simulink model "task1"  (R2018a)
settings: Solver=ode1  StartTime=0.0  StopTime=inf  FixedStep=0.01  RelTol=1e-3
settings Model: Creator=richardkong  LastModifiedBy=richardkong

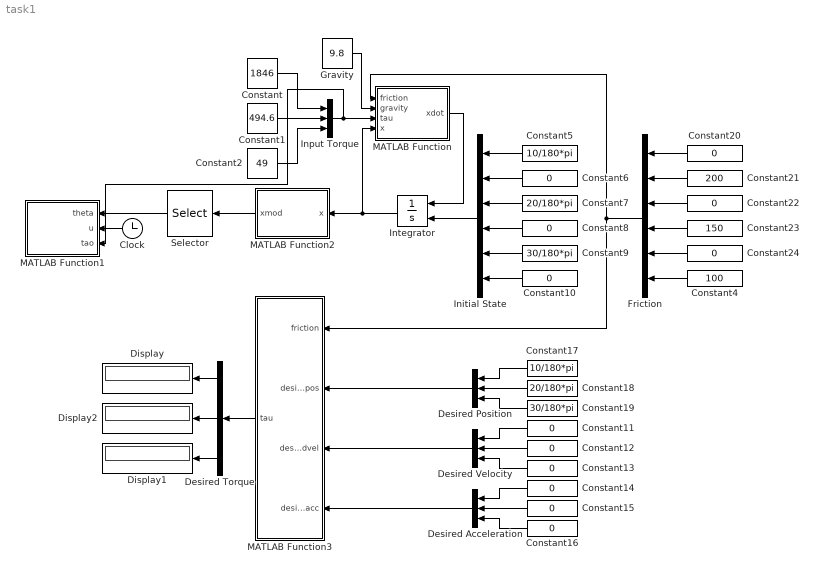
== system task1 ==
  Clock : Clock
  Constant : Constant  Value=1846
  Constant1 : Constant  Value=494.6
  Constant{6,8,10..16,20,22,24} (12 alike) : Constant  Value=0
  Constant17 : Constant  Value=10/180*pi
  Constant18 : Constant  Value=20/180*pi
  Constant19 : Constant  Value=30/180*pi
  Constant2 : Constant  Value=49
  Constant21 : Constant  Value=200
  Constant23 : Constant  Value=150
  Constant4 : Constant  Value=100
  Constant5 : Constant  Value=10/180*pi
  Constant7 : Constant  Value=20/180*pi
  Constant9 : Constant  Value=30/180*pi
  Desired Acceleration : BusCreator  Inputs=3
  Desired Position : BusCreator  Inputs=3
  Desired Torque : Demux  Outputs=3
  Desired Velocity : BusCreator  Inputs=3
  Display : Display
  Display1 : Display
  Display2 : Display
  Friction : BusCreator  Inputs=6
  Gravity : Constant  Value=9.8
  Initial State : BusCreator  Inputs=6
  Input Torque : BusCreator  Inputs=3
  Integrator : Integrator  InitialConditionSource=external  InitialCondition=[1/18*pi;0;1/9*pi;0;1/6*pi;0]
  MATLAB Function : MATLAB Function  TreatAsAtomicUnit=on
  MATLAB Function1 : MATLAB Function  TreatAsAtomicUnit=on
  MATLAB Function2 : MATLAB Function  TreatAsAtomicUnit=on
  MATLAB Function3 : MATLAB Function  TreatAsAtomicUnit=on
  Selector : Selector  InputPortWidth=6  IndexOptions=Index vector (dialog)  Indices=[1 3 5]  OutputSizes=1
  wires:
  Integrator/1 -> MATLAB Function2/1(x), MATLAB Function/4(x)
  Selector/1 -> MATLAB Function1/1(theta)
  MATLAB Function/1(xdot) -> Integrator/1
  Constant1/1 -> Input Torque/2
  Constant2/1 -> Input Torque/3
  Constant/1 -> Input Torque/1
  Input Torque/1 -> MATLAB Function1/3(tao), MATLAB Function/3(tau)
  Gravity/1 -> MATLAB Function/2(gravity)
  MATLAB Function2/1(xmod) -> Selector/1
  Friction/1 -> MATLAB Function3/1(friction), MATLAB Function/1(friction)
  Initial State/1 -> Integrator/2
  Constant5/1 -> Initial State/1
  Constant10/1 -> Initial State/6
  Constant9/1 -> Initial State/5
  Constant8/1 -> Initial State/4
  Constant7/1 -> Initial State/3
  Constant6/1 -> Initial State/2
  Constant11/1 -> Desired Velocity/1
  Constant13/1 -> Desired Velocity/3
  Constant12/1 -> Desired Velocity/2
  Constant15/1 -> Desired Acceleration/2
  Constant16/1 -> Desired Acceleration/3
  Constant14/1 -> Desired Acceleration/1
  Constant18/1 -> Desired Position/2
  Constant19/1 -> Desired Position/3
  Constant17/1 -> Desired Position/1
  MATLAB Function3/1(tau) -> Desired Torque/1
  Desired Position/1 -> MATLAB Function3/2(desiredpos)
  Desired Velocity/1 -> MATLAB Function3/3(desiredvel)
  Desired Acceleration/1 -> MATLAB Function3/4(desiredacc)
  Desired Torque/3 -> Display1/1
  Desired Torque/2 -> Display2/1
  Desired Torque/1 -> Display/1
  Constant20/1 -> Friction/1
  Constant23/1 -> Friction/4
  Constant22/1 -> Friction/3
  Constant21/1 -> Friction/2
  Constant4/1 -> Friction/6
  Constant24/1 -> Friction/5
  Clock/1 -> MATLAB Function1/2(u)

== matlab function task1/MATLAB Function1 ==
  data: theta input; u input; tao input
function animate(theta,u,tao)
%#codegen
coder.extrinsic('saveas');
coder.extrinsic('num2str');
u = int16( u / 0.01) + 1;
theta1 = theta(1);
theta2 = theta(2);
theta3 = theta(3);
%hold off
T_0 = eye(4);
hold off
l1 = 4;
l2 = 3;
l3 = 2;
point1=[[0,0,0];[4,0,0]];
point2 = [[0,0,0];[3,0,0]];
point3 = [[0,0,0];[2,0,0]];

T_01 = [cos(theta1) -sin(theta1) 0 0; sin(theta1) cos(theta1) 0 0; 0 0 1 0; 0 0 0 1];
T_12 = [cos(theta2) -sin(theta2) 0 l1; sin(theta2) cos(theta2) 0 0; 0 0 1 0; 0 0 0 1];
T_23 = [cos(theta3) -sin(theta3) 0 l2; sin(theta3) cos(theta3) 0 0; 0 0 1 0; 0 0 0 1];

point1 = [point1 [1;1]];
point2 = [point2 [1;1]];
point3 = [point3 [1;1]];
     
point1 = (T_0 * T_01 * point1')';
       
point2 = (T_0 * T_01 * T_12 * point2')';

point3 = (T_0 * T_01 * T_12 * T_23 * point3')';

plot(point1(:,1),point1(:,2));
hold on
plot(point2(:,1),point2(:,2));
grid on
plot(point3(:,1),point3(:,2));
grid on
axis([-15 15 -15 15 -15 15]);
xlabel('X');
ylabel('Y');
title(['With Torque 1 = ',num2str(tao(1)),', Torque 2 = ',num2str(tao(2)),', Torque 3 = ',num2str(tao(3)),', With Gravity']);
if rem(u, 10) == 1
    saveas(gcf,['/Users/richardkong/Desktop/Robotics/Final/Joint3/',num2str(u,'%04d')],'png');
end
end

== matlab function task1/MATLAB Function ==
  data: friction input; gravity input; tau input; xdot output; x input
function xdot = Dynamic(friction, gravity, tau, x)
%#codegen
theta1 = x(1);
theta_1 = x(2);
theta2 = x(3);
theta_2 = x(4);
theta3 = x(5);
theta_3 = x(6);

f_1 = friction(2);
f_2 = friction(4);
f_3 = friction(6);

g = gravity;
tau1 = tau(1);
tau2 = tau(2);
tau3 = tau(3);

m1 = 20;
m2 = 15;
m3 = 10;
l1 = 4;
l2 = 3;
l3 = 2;
Izz1 = 0.5;
Izz2 = 0.2;
Izz3 = 0.1;

M11 = m3 * (l1^2 + l2^2 + l3^2/4 + 2*l1*l2*cos(theta2) + l2*l3*cos(theta3) + l1*l3*cos(theta2 + theta3)) + m2 * (l1^2 + l2^2/4 + l1*l2*cos(theta2)) + m1 * l1^2/4 + Izz1 + Izz2 + Izz3;
M12 = m3 * (l2^2 + l3^2/4 + l1*l2*cos(theta2) + l2*l3*cos(theta3) + l1*l3/2*cos(theta2 + theta3)) + m2 * (l2^2/4 + l1*l2/2*cos(theta2)) + Izz2 + Izz3;
M13 = m3 * (l3^2/4 + l2*l3/2*cos(theta3) + l1*l3/2*cos(theta2 + theta3)) + Izz3;
M21 = M12;
M22 = m3 * (l2^2 + l3^2/4 + l2*l3*cos(theta3)) + m2 * l2^2/4 + Izz2 + Izz3;
M23 = m3 * (l3^2/4 + l2*l3/2*cos(theta3)) + Izz3;
M31 = M13;
M32 = M23;
M33 = m3 * l3^2/4 + Izz3;

C12 = m3 * (-l1*l2*sin(theta2) - l1*l3/2*sin(theta2 + theta3)) + m2 * (-l1*l2/2*sin(theta2));
C21 = -C12;
C13 = m3 * (-l2*l3/2*sin(theta3) - l1*l3/2*sin(theta2 + theta3));
C31 = -C13;
C23 = m3 * (-l2 * l3 / 2 * sin(theta3));
C32 = -C23;

B11 = 2 * (m3 * (-l1*l2*sin(theta2)-l1*l3/2*sin(theta2 + theta3)) + m2 * (-l1 * l2/2 * sin(theta2)));
B12 = 2 * (m3 * (-l2*l3/2*sin(theta3)-l1*l3/2*sin(theta2 + theta3)));
B13 = B12;
B22 = -2 * (m3 * l2 * l3 / 2 * sin(theta3));
B23 = B22;
B31 = -1 * B23;

G1 = cos(theta1)*l1/2*m1*g + (cos(theta1+theta2)*l2/2+cos(theta1)*l1)*m2*g + (cos(theta1 + theta2 + theta3)*l3/2 + cos(theta1 + theta2)*l2 + cos(theta1)*l1) * m3*g;
G2 = cos(theta1+theta2)*l2/2*m2*g + (cos(theta1 + theta2 + theta3)*l3/2 + cos(theta1 + theta2)*l2) * m3*g;
G3 = cos(theta1 + theta2 + theta3)*l3/2 * m3 * g;

M = [M11 M12 M13; M21 M22 M23; M31 M32 M33];
C = [0 C12 C13; C21 0 C23; C31 C32 0];
B = [B11 B12 B13; 0 B22 B23; B31 0 0];
G = [G1; G2; G3];

ans = [tau1-f_1*theta_1;tau2-f_2*theta_2;tau3-f_3*theta_3] - C * [theta_1^2;theta_2^2;theta_3^2] - B * [theta_1 * theta_2;theta_1 * theta_3;theta_2 * theta_3] - G;
E = inv(M) * ans;
theta_11 = E(1);
theta_22 = E(2);
theta_33 = E(3);

xdot = [theta_1; theta_11; theta_2; theta_22; theta_3; theta_33];
end

== matlab function task1/MATLAB Function2 ==
  data: x input; xmod output
function xmod = module(x)
q1 = x(1);
q2 = x(3);
q3 = x(5);
q1 = atan2(sin(q1), cos(q1));
q2 = atan2(sin(q2), cos(q2));
q3 = atan2(sin(q3), cos(q3));
xmod = [q1;x(2);q2;x(4);q3;x(6)];

== matlab function task1/MATLAB Function3 ==
  data: friction input; tau output; desiredpos input; desiredvel input; desiredacc input
function tau = Torque(friction, desiredpos, desiredvel, desiredacc)
%#codegen
theta1 = desiredpos(1);
theta2 = desiredpos(2);
theta3 = desiredpos(3);
theta_1 = desiredvel(1);
theta_2 = desiredvel(2);
theta_3 = desiredvel(3);
theta_11 = desiredacc(1);
theta_22 = desiredacc(2);
theta_33 = desiredacc(3);

f_1 = friction(2);
f_2 = friction(4);
f_3 = friction(6);

E = [theta_11; theta_22; theta_33];

g = 9.8;

m1 = 20;
m2 = 15;
m3 = 10;
l1 = 4;
l2 = 3;
l3 = 2;
Izz1 = 0.5;
Izz2 = 0.2;
Izz3 = 0.1;

M11 = m3 * (l1^2 + l2^2 + l3^2/4 + 2*l1*l2*cos(theta2) + l2*l3*cos(theta3) + l1*l3*cos(theta2 + theta3)) + m2 * (l1^2 + l2^2/4 + l1*l2*cos(theta2)) + m1 * l1^2/4 + Izz1 + Izz2 + Izz3;
M12 = m3 * (l2^2 + l3^2/4 + l1*l2*cos(theta2) + l2*l3*cos(theta3) + l1*l3/2*cos(theta2 + theta3)) + m2 * (l2^2/4 + l1*l2/2*cos(theta2)) + Izz2 + Izz3;
M13 = m3 * (l3^2/4 + l2*l3/2*cos(theta3) + l1*l3/2*cos(theta2 + theta3)) + Izz3;
M21 = M12;
M22 = m3 * (l2^2 + l3^2/4 + l2*l3*cos(theta3)) + m2 * l2^2/4 + Izz2 + Izz3;
M23 = m3 * (l3^2/4 + l2*l3/2*cos(theta3)) + Izz3;
M31 = M13;
M32 = M23;
M33 = m3 * l3^2/4 + Izz3;

C12 = m3 * (-l1*l2*sin(theta2) - l1*l3/2*sin(theta2 + theta3)) + m2 * (-l1*l2/2*sin(theta2));
C21 = -C12;
C13 = m3 * (-l2*l3/2*sin(theta3) - l1*l3/2*sin(theta2 + theta3));
C31 = -C13;
C23 = m3 * (-l2 * l3 / 2 * sin(theta3));
C32 = -C23;

B11 = 2 * (m3 * (-l1*l2*sin(theta2)-l1*l3/2*sin(theta2 + theta3)) + m2 * (-l1 * l2/2 * sin(theta2)));
B12 = 2 * (m3 * (-l2*l3/2*sin(theta3)-l1*l3/2*sin(theta2 + theta3)));
B13 = B12;
B22 = -2 * (m3 * l2 * l3 / 2 * sin(theta3));
B23 = B22;
B31 = -1 * B23;

G1 = cos(theta1)*l1/2*m1*g + (cos(theta1+theta2)*l2/2+cos(theta1)*l1)*m2*g + (cos(theta1 + theta2 + theta3)*l3/2 + cos(theta1 + theta2)*l2 + cos(theta1)*l1) * m3*g;
G2 = cos(theta1+theta2)*l2/2*m2*g + (cos(theta1 + theta2 + theta3)*l3/2 + cos(theta1 + theta2)*l2) * m3*g;
G3 = cos(theta1 + theta2 + theta3)*l3/2 * m3 * g;

M = [M11 M12 M13; M21 M22 M23; M31 M32 M33];
C = [0 C12 C13; C21 0 C23; C31 C32 0];
B = [B11 B12 B13; 0 B22 B23; B31 0 0];
G = [G1; G2; G3];

tau = M * E + C * [theta_1^2;theta_2^2;theta_3^2] + B * [theta_1 * theta_2;theta_1 * theta_3;theta_2 * theta_3] + G;
tau = tau + [theta_1 * f_1;theta_2 * f_2;theta_3 * f_3];
end
